simulink model "BATTERYLESS_SOLAR_INVERTER_DRIVE"  (R2021a)
settings: Solver=ode15s  StartTime=0.0  StopTime=inf  FixedStep=.00001  MaxStep=.00001  RelTol=1e-3  EnableMultiTasking=on
undefined symbols (not defined in the file): Capacitor, dEgdT, EgRef, gcbh, k1, Rsh_array5pc, Run, sps_rtmsupport, Start, Tref_K, VT_ref
libraries: fl_lib x7, spsCurrentMeasurementLib x6, nesl_utility x6, sh_lib x5, spsSeriesRLCBranchLib x5, spsIGBTDiodeLib x4, spsVoltageMeasurementLib x4, pid_lib x3, spsPVarrayModel x3, simulink x3, spsControlledCurrentSourceLib x2, spsRMSLib x2
(part 1 of 5)
settings Model: NumberOfSteps=100000000  Creator=Mahbubur Rahman  LastModifiedBy=This PC
settings SolverCC: AlgebraicLoopSolver=LineSearch
settings DataIOCC: LimitDataPoints=on  SaveFormat=Array  ReturnWorkspaceOutputs=off
settings OptimizationCC: LifeSpan=inf
settings DebuggingCC: SFUnexpectedBacktrackingDiag=warning  SFNoUnconditionalDefaultTransitionDiag=warning  SFExecutionAtInitializationDiag=none  SFMachineParentedDataDiag=warning  ArithmeticOperatorsInVariantConditions=warning
settings HardwareCC: ProdBitPerPointer=32  ProdBitPerSizeT=32  ProdBitPerPtrDiffT=32  ProdLargestAtomicFloat=None  ProdIntDivRoundTo=Undefined  ProdEndianess=Unspecified  ProdWordSize=32  ProdHWDeviceType=32-bit Generic
settings ModelReferenceCC: PropagateSignalLabelsOutOfModel=off
settings SFSimCC: SimUseLocalCustomCode=off  CustomCodeUndefinedFunction=UseInterfaceOnly
settings RTWCC: RTWUseLocalCustomCode=off
settings CodeAppCC: StateflowObjectComments=on
settings GRTTargetCC: TargetLangStandard=C89/C90 (ANSI)
settings ConfigComp: CovMetricSettings=dw  CovSaveCumulativeToWorkspaceVar=on  CovSaveSingleToWorkspaceVar=on  CovExternalEMLEnable=off
settings SimscapeCC: SimscapeNormalizeSystem=off

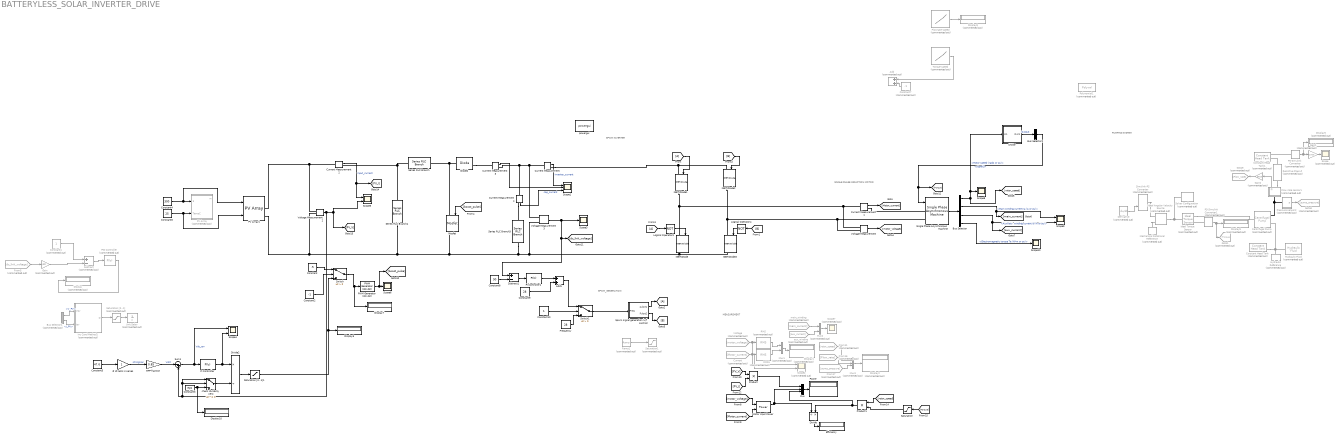
== system BATTERYLESS_SOLAR_INVERTER_DRIVE ==
  note: SPWM INVERTER
  note: PUMPING SYSTEM
  note: SINGLE PHASE INDUCTION MOTOR
  note: MEASUREMENT
  note: SPWM_GENERATION
  # of cells in series : Gain
  Add : Sum  Commented=on
  Add1 : Sum
  Bus Selector : BusSelector  OutputSignals="Mechanical.Rotor speed (rad/s or pu),Stator measurements.Main winding current Ia (A or pu),Stator measurements.Auxiliary  winding current Ib (A or pu),Mechanical.Electromagnetic torque Te (N*m or pu)"
  Bus Selector1 : BusSelector  Commented=on  OutputSignals=V_PV,I_PV
  Bus Selector2 : BusSelector  OutputSignals=signal3
  Centrifugal Pump : sh_lib/Pumps and Motors/Centrifugal Pump  Commented=on  mdl_type=1  c_1=326.8 Pa/(kg/m^3)  c_2=3.104e+4 Pa*s/kg  c_3=1.097e+7 Pa*s^2/(kg*m^3)  c_4=2.136e+5 Pa*s^2/(kg*m^3)  c_f=0.8  design_del=130 lpm  ref_velocity=1500 rpm  ref_density=1000 kg/m^3  leak_resistance=1e+8 Pa/(m^3/s)  T_const=0.1 N*m  trq_press_coeff=1e-6 N*m/Pa  pump_del_1D=[ 0 28 90 130 154 182 ] lpm  press_diff_1D=[ 2.6 2.4 2 1.6 1.2 0.8 ] bar  pump_del_power_1D=[ 0 20 40 60 80 100 120 140 160 ] lpm  power_1D=[ 220 280 310 360 390 420 480 500 550 ] W  pump_vel_2D=[ 3.2e+3 3.3e+3 3.4e+3 3.5e+3 ] rpm  pump_del_2D=[ 0 50 100 150 200 250 300 350 ] lpm  press_diff_2D=[ 8.300000000000001 8.800000000000001 9.300000000000001 9.9; 7.8 8.300000000000001 8.800000000000001 9.4; 7.2 7.6 8.199999999999999 8.699999999999999; 6.5 7 7.5 8; 5.6 6.1 6.6 7.1; 4.7 5.2 5.7 6.2; 3.4 4 4.4 4.9; 2.3 2.7 3.4 3.6 ] bar  pump_del_power_2D=[ 0 50 100 150 200 250 300 350 ] lpm  power_2D=[ 1.223e+3 1.341e+3 1.467e+3 1.6e+3; 1.414e+3 1.551e+3 1.696e+3 1.85e+3; 1.636e+3 1.794e+3 1.962e+3 2.14e+3; 1.941e+3 2.129e+3 2.326e+3 2.54e+3; 2.224e+3 2.439e+3 2.66e+3 2.91e+3; 2.453e+3 2.691e+3 2.947e+3 3.21e+3; 2.757e+3 3.024e+3 3.307e+3 3.608e+3; 2.945e+3 3.23e+3 3.533e+3 3.854e+3 ] W  omega_threshold=1e-9 rad/s  interp_method=2  extrap_method=1
      settings: SourceProductBaseCode=SH  InternalSimscapePortConfiguration="{\"Bottom\":[],\"Left\":[{\"id\":\"S\",\"label\":\"S\",\"type\":\"foundation.mechanical.rotational.rotational\"}],\"Right\":[{\"id\":\"P\",\"label\":\"P\",\"type\":\"foundation.hydraulic.hydraulic\"},{\"id\":\"T\",\"label\":\"T\",\"type\":\"foundation.hydraulic.hydraulic\"}],\"Top\":[]}"
  Chiller : Subsystem
  Constant : Constant  Value=.5
  Constant Head Tank : sh_lib/Low-Pressure Blocks/Constant Head Tank  Commented=on  press=0 Pa  fluid_level=1 m  pipe_diam=10 cm  loss_coeff=1.2  g=9.80665 m/s^2  volume_specify=on  volume_priority=High  volume=10000000 m^3  volume_nominal_specify=off  volume_nominal_unit=m^3  volume_nominal_value=1
      settings: SourceProductBaseCode=SH  InternalSimscapePortConfiguration="{\"Bottom\":[],\"Left\":[],\"Right\":[{\"id\":\"V\",\"label\":\"V\",\"type\":\"output\"},{\"id\":\"T\",\"label\":\"T\",\"type\":\"foundation.hydraulic.hydraulic\"}],\"Top\":[]}"
  Constant Head Tank1 : sh_lib/Low-Pressure Blocks/Constant Head Tank  Commented=on  press=0 Pa  fluid_level=0 m  pipe_diam=0.02 m  loss_coeff=1.2  g=9.80665 m/s^2  volume_specify=on  volume_priority=High  volume=0 m^3  volume_nominal_specify=off  volume_nominal_unit=m^3  volume_nominal_value=1
      settings: SourceProductBaseCode=SH  InternalSimscapePortConfiguration="{\"Bottom\":[],\"Left\":[],\"Right\":[{\"id\":\"V\",\"label\":\"V\",\"type\":\"output\"},{\"id\":\"T\",\"label\":\"T\",\"type\":\"foundation.hydraulic.hydraulic\"}],\"Top\":[]}"
  Constant1 : Constant  Commented=on
  Constant10 : Constant
  Constant2 : Constant  Value=-1
  Constant3 : Constant  Value=eps
  Constant4 : Constant  Value=300
  Constant5 : Constant  Value=47.6
  Constant6 : Constant  Value=25
  Constant7 : Constant  Commented=on  Value=.1
  Constant8 : Constant  Value=90
  Constant9 : Constant  Value=28
  Current : From  Commented=on  GotoTag=Motor_current
  Current Measurement{,1..4} (5 alike) : spsCurrentMeasurementLib/Current Measurement  PhasorSimulation=off  OutputType=Complex  PSBequivalent=0
  Derivative : Derivative  Commented=on
  Diode2 : spsDiodeLib/Diode  Ron=0.001  Lon=0  Vf=0.8  IC=0  UseSnubber=0  Rs=500  Cs=250e-9  Measurements=on
  Display{,1..2,6,8..9} (6 alike) : Display  Commented=on
  Display10 : Display
  Display5 : Display
  Display7 : Display
  Divide : Product  Inputs=/*
  Divide2 : Product  Inputs=*/
  "Efficiency " : Display
  Flow rate sensor1 : Subsystem  Commented=on
      mask Display:
      | plot([141.749396522682;150.34840079814;159.942662684676;170.439784195567;181.738672312351;193.730512565863;206.299816979056;219.32553627935;232.6822256693;246.241252928572;259.872037212541;273.443306617208;286.824362399395;299.886337677091;312.503438487969;324.554155254012;335.922432985171;346.498788952362;356.181367065997;364.876918805806;365.635077753444], [311.772266015396;301.195910048205;291.51333193457;282.817780194761;275.192997745505;268.712415409918;263.438444738539;259.421876951977;256.701393793698;255.303195003683;255.240746000613;256.514648202526;259.112633234831;263.009681081464;268.168261041319;274.538693169416;282.05962672193;290.658630997388;300.252892883924;310.750014394814;311.772273468441])
      | plot([141.699510299516;151.06208312931;161.43851880176;172.728886569004;184.8244540175;197.608734220609;210.958607571377;224.745507491653;238.836658598519;253.096355403808;267.387269232142;281.571770771148;295.513255516966;309.077459350303;322.133751573297;334.556392954544;346.225746666638;357.029430454211;366.863398936497;369.389910236765], [142.635753971168;153.439437758742;163.273406241027;172.042952925747;179.663622284404;186.062023105194;191.17653529049;194.957903292072;197.369710468977;198.388729799666;198.005147570929;196.222657889318;193.058427104875;188.542928489797;182.719648764172;175.644669295084;167.3861260024;158.023553172606;147.647117500155;144.622762828085])
      | plot([255.112000578148;241.220263814025;227.462288078042;213.97057019741;200.875042790642;188.30182294541;176.371997642044;165.200457619721;154.894790915842;145.554246734416;137.268779621969;130.118183156093;124.171321489666;119.485466151423;116.10574448982;114.064705072001;113.382004223305;114.064216726109;116.104772501074;119.484019880607;124.169414865158;130.115834539728;137.266011632208;145.551086028513;154.891267933124;165.196606288436;176.367855052617;188.297428993243;200.870439791896;213.965802481478;227.457401560637;241.21530555498;255.107018328207;268.99875509233;282.756730828313;296.248448708946;309.343976115713;321.917195960945;333.847021264311;345.018561286634;355.324227990513;364.66477217194;372.950239284386;380.100835750262;386.047697416689;390.733552754932;394.113274416535;396.154313834354;396.83701468305;396.154802180246;394.114246405281;390.734999025748;386.049604041197;380.103184366627;372.953007274147;364.667932877842;355.327750973232;345.022412617919;333.851163853738;321.921589913113;309.34857911446;296.253216424877;282.761617345719;269.003713351376;255.112000578149;255.112000578148;255.112000578148], [85.0365031729522;85.7187156757559;87.7592714507213;91.138518830254;95.823913814805;101.770333489375;108.920510581855;117.20558497816;126.54576688277;136.851105238083;148.022354002264;159.951927942889;172.524938741542;185.620301431125;199.111900510283;212.869804504627;226.761517277854;240.653254041976;254.41122977796;267.902947658592;280.99847506536;293.571694910592;305.501520213958;316.673060236281;326.97872694016;336.319271121586;344.604738234033;351.755334699909;357.702196366336;362.388051704579;365.767773366182;367.808812784001;368.491513632697;367.809301129893;365.768745354927;362.389497975395;357.704102990844;351.757683316273;344.607506223793;336.322431827489;326.982249922878;316.676911567566;305.505662803384;293.576088862759;281.003078064106;267.907715374523;254.416116295365;240.658212301022;226.766499527795;212.874762763672;199.116787027689;185.625069147057;172.529541740289;159.956321895057;148.026496591691;136.854956569369;126.54928986549;117.208745684063;108.923278571616;101.77268210574;95.8258204393135;91.1399651010703;87.7602434394666;85.7192040216476;85.0365031729522;85.0365031729522;85.0365031729522])
      | plot([113.382004201412;56.6910021007061], [226.764008402824;226.764008402824])
      | plot([396.837014704943;453.528016805649;450.693466700613], [226.764008402824;226.764008402824;226.764008402824])
      | plot([510.219018906355;0;0;510.219018906355;510.219018906355], [510.219018906355;510.219018906355;0;0;510.219018906355])
      | ;color('red');
      | port_label('LConn', 1,'A')
      | port_label('RConn', 1,'B')
  Flowrate-speed : Lookup_n-D  Commented=on  NumberOfTableDimensions=1  BreakpointsForDimension1=[0,0.755267129742124,3.94138541604345,4.4414537006491,7.53165396046033,8.07857474382879,11.1492675042464,11.7097698895216,14.7704457545395,15.3535511531923,18.3855000155405,19.023728886058,21.9935096148579,22.730877418348,25.6001483967937,26.4827517809723,29.2158883182174,30.283293810304,32.8535466181619,34.1309377359887,36.5253360532606,38.0175805064918,40.2403035353047,41.9296372251585,44.0030919829905,45.8517320387111,47.8142383144331,49.7719032061007,51.6711955449403,53.6857443686728,55.5689445180788,57.5970867055065,59.5000308517515,61.5149482189319,63.4551949595903,65.4488392003123,67.4256256724198,69.4050214570267,71.4059609943714,73.3849875878053,75.3957115737105,77.3860986863011,79.3978365933288,81.4038216961908,83.4156531732883,85.434477767689,87.4503871026008,89.4768321784884,91.5007566875217,93.5315546937149,95.5585766457447,96.3816078917583,97.1583244877688,97.5553159469706,98.5109556896585,98.942464160912,99.7574872364738,100.421283742859,101.07463594914,101.853778607577,102.481394416513,103.244540211763,103.936132120085,104.652018040325,105.393813499244,106.098856898837,106.848483926202,107.575303616505,108.316989524379,109.066251289772,109.809284913161,110.568387478049,111.323498843144,112.086670722946,112.854874120687,113.624667016258,114.40227865717,115.182041566037,115.967331307467,116.757422142148,117.551245116694,118.350605567398,119.153989085531,119.962222924494,120.775257982183,121.592720182895,122.415140879025,123.242160081895,124.073946581288,124.910563281961,125.751889693993,126.598080049304,127.449074625766,128.304901941835,129.165610952387,130.031176064865,130.90164360049,131.777020135967,132.657315099945,133.542556003384,134.432747653115,135.327908481052,136.228053440758,137.133192405713,138.043341260578,138.958510842986,139.87871256473,140.803958431303,141.734257902805,142.669621071515,143.610056994698,144.555573622054,145.50617867552,146.461878717645,147.422679531354,148.38858614358,149.359602511583,150.335731721296,151.316975860531,152.30333593763,153.294811920063,154.291402633151,155.293105725223,156.299917638184,157.311833536082,158.328847265387,159.350951303764,160.378136699555,161.410393021146,162.447708298236,163.490068961237,164.537459782067,165.589863810492,166.647262309323,167.709634688423,168.776958435952,169.849206150296,170.923006726351,171.99390815586,173.062561647706,174.129436376986,175.194952410275,176.259419194953,177.323066108992,178.386056645792,179.448487812122,180.510448409105,181.572036759616,182.633352690859,183.694493078604,184.755547514223,185.816595543058,186.877705530537,187.93893392239,189.000325086927,190.061911650665,191.123715182272,192.185758808865,193.248076932833,194.310686031143,195.373582867113,196.436747999436,197.500148410283,198.563739469472,199.627466414353,200.6912655164,201.755065006481,202.818785812219,203.882342160934,204.945642078165,206.008587802641,207.071076137412,208.132998750829,209.19424243718,210.254689345506,211.31421718332,212.372699400335,213.430005356484,214.486000477789,215.540546402947,216.59350112303,217.644719116346,218.694051480172,219.741346060803,220.786448265843,221.829205247654,222.869465287781,223.907074945561,224.941879059511,225.973720793947,227.002441697075,228.027881769757,229.049879541202,230.06827215286,231.08289545147,232.093584090637,233.100171640738,234.102490707285,235.100373057609,236.093649755654,237.082151304686,238.065707797705,239.044149075298,240.017304890621,240.985005081183,241.947079747063,242.903359435172,243.853675329111,244.797859444178,245.735744827019,246.6671657594,247.591957965548,248.50995882248,249.421007572714,250.32494553873,251.221616338524,252.110866101598,252.99254368468,253.86650088649,254.732592660822,255.590677327237,256.440616778643,257.28227668503,258.115526692641,258.940240617881,259.756296635252,260.563577458626,261.36197051521,262.15136811153,262.931667590861,263.702771481481,264.464587635229,265.217029355844,265.960015516618,266.693470666946,267.417325127393,268.131515072948 ...(+2740 chars)]  Table=[-2.49551596944865e-05,-2.49549147032931e-05,-2.49484380819495e-05,-2.49466297780723e-05,-2.49306026044872e-05,-2.49269113638027e-05,-2.49013121298883e-05,-2.48957594374241e-05,-2.48605733783786e-05,-2.48529407394126e-05,-2.480845080358e-05,-2.47980468706096e-05,-2.47449474830391e-05,-2.47305343651049e-05,-2.46699144918519e-05,-2.46497599560278e-05,-2.45829899241857e-05,-2.45550454605781e-05,-2.4483588126165e-05,-2.44457860626406e-05,-2.43709488524717e-05,-2.4321576461125e-05,-2.42442283291449e-05,-2.41822885846768e-05,-2.41025904730598e-05,-2.40280252732902e-05,-2.3945261125573e-05,-2.38589273594273e-05,-2.37715467273756e-05,-2.36749127185171e-05,-2.35808557660346e-05,-2.34754954913822e-05,-2.33727420647344e-05,-2.32597916187635e-05,-2.31469168499245e-05,-2.30266881082214e-05,-2.29031464467343e-05,-2.27750597666361e-05,-2.2641042316839e-05,-2.25039266552064e-05,-2.23598806835534e-05,-2.22124971407542e-05,-2.20585923775605e-05,-2.19000743546397e-05,-2.17359181246507e-05,-2.1565859764012e-05,-2.13905911859891e-05,-2.12087761130309e-05,-2.10214053780375e-05,-2.08274350068393e-05,-2.06276763071934e-05,-2.0544708332486e-05,-2.04655251262348e-05,-2.04246356753725e-05,-2.03253729585894e-05,-2.02799850665838e-05,-2.01935869076218e-05,-2.01223720606876e-05,-2.0051575766443e-05,-1.99662400392406e-05,-1.98967224332311e-05,-1.98113241626112e-05,-1.97330411005835e-05,-1.96511354611788e-05,-1.95653090927907e-05,-1.94828100497838e-05,-1.93941129044323e-05,-1.930711683095e-05,-1.92173274242324e-05,-1.91255616966952e-05,-1.90334902991678e-05,-1.89383183557908e-05,-1.88425118100022e-05,-1.87445187791029e-05,-1.86446778313321e-05,-1.85434008084471e-05,-1.84398264912865e-05,-1.83346618978678e-05,-1.82274108267435e-05,-1.81181212626141e-05,-1.80068930196575e-05,-1.78934217523123e-05,-1.77778671345495e-05,-1.76600553422711e-05,-1.75399336130264e-05,-1.74174959571178e-05,-1.72925985157255e-05,-1.71652278871072e-05,-1.70352876409391e-05,-1.69026932578763e-05,-1.67673856293163e-05,-1.66292577592988e-05,-1.64882325221105e-05,-1.63442138742351e-05,-1.61970969820236e-05,-1.60467841169421e-05,-1.58931592194649e-05,-1.57361065042925e-05,-1.55755026505602e-05,-1.54112132679794e-05,-1.52430996363834e-05,-1.50710112360041e-05,-1.48947879668254e-05,-1.47142594923345e-05,-1.45292418833336e-05,-1.43395384646981e-05,-1.41449371791413e-05,-1.39452088002874e-05,-1.37401055714289e-05,-1.3529358168955e-05,-1.33126733045148e-05,-1.30897305185023e-05,-1.28601781590027e-05,-1.26236290618357e-05,-1.2379655032421e-05,-1.21277802855679e-05,-1.18674735560113e-05,-1.15981382649136e-05,-1.13191004222428e-05,-1.10295934435953e-05,-1.07287388420761e-05,-1.04155214338913e-05,-1.00887569265338e-05,-9.74704884365562e-06,-9.38873016383182e-06,-9.01178241294498e-06,-8.61372054797799e-06,-8.19142403767303e-06,-7.74087967555675e-06,-7.25677202315763e-06,-6.73179360231919e-06,-6.15539614279133e-06,-5.51130007439783e-06,-4.7717907156445e-06,-3.88146314991264e-06,-2.68623152633747e-06,1.25160354243976,63.3665222781476,119.652343191978,171.805480489557,220.121632951326,265.161240746742,307.558847273221,347.779385477827,386.506555351731,424.189316880001,460.699631721232,495.965114144391,529.961450844176,562.700870365115,594.221157898742,624.576449882164,653.830146784885,682.049771150408,709.303441601163,735.657585852094,761.16848729897,785.802243671772,809.653445329318,832.838381314817,855.448629118332,877.557723581626,899.225678657012,920.502149201249,941.428700665877,962.040476456674,982.367447082747,1002.43536223163,1022.26648778397,1041.88018419473,1061.2933659522,1080.52087066198,1099.57575853552,1118.46955763738,1137.21246641651,1155.81352226635,1174.28074282024,1192.62124518544,1210.84134719072,1228.94665386502,1246.94213171072,1264.83217282952,1282.62065056483,1300.31096801495,1317.90063638302,1335.37823672611,1352.74020310878,1369.98343411612,1387.10503185905,1404.1022908572,1420.97268689659,1437.7138659716,1454.32363335805,1470.79994293292,1487.14088683621,1503.3446855316 ...(+3432 chars)]  InternalRulePriority=Speed  RndMeth=Simplest  InputSameDT=on
  "Frequency " : Constant  Value=28
  From11 : From  Commented=on  GotoTag=rotor_speed
  From16 : From  Commented=on  GotoTag=Flow_rate
  From17 : From  Commented=on  GotoTag=pump_pressure
  From5 : From  Commented=on  GotoTag=dc_link_voltage
  Gain : Gain  Commented=on  Gain=1/80
  Gain1 : Gain  Commented=on  Gain=1000
  Gain2 : Gain  Commented=on  Gain=36e5
  Goto1 : Goto  Commented=on  GotoTag=Torque
  Goto8 : Goto  Commented=on  GotoTag=pump_pressure
  Goto9 : Goto  Commented=on  GotoTag=Flow_rate
  Hydraulic Fluid : sh_lib/Hydraulic Utilities/Hydraulic Fluid  Commented=on  DataSource=1  SelFluid=24  SysTemp=60  TrapAir=0.005  ViscDerFactor=1  range_error=2
  Hydraulic Reference : fl_lib/Hydraulic/Hydraulic Elements/Hydraulic Reference  Commented=on
  IGBT/Diode{,1..3} (4 alike) : spsIGBTDiodeLib/IGBT//Diode  Ron=1e-3  Rs=1e5  Cs=inf  Measurements=on
  Ideal Angular Velocity Source : fl_lib/Mechanical/Mechanical Sources/Ideal Angular Velocity Source  Commented=on
  Ideal Torque Sensor : fl_lib/Mechanical/Mechanical Sensors/Ideal Torque Sensor  Commented=on
  Inc Cond Method1 : Stateflow chart  Commented=on  TreatAsAtomicUnit=on
  Logical Operator3 : Logic  Operator=NOT  AllPortsSameDT=off  OutDataTypeStr=boolean
  Logical Operator4 : Logic  Operator=NOT  AllPortsSameDT=off  OutDataTypeStr=boolean
  MPP fraction : Gain  Gain=0.85
  Mechanical Rotational Reference : fl_lib/Mechanical/Rotational Elements/Mechanical Rotational Reference  Commented=on
  Mosfet : spsMosfetLib/Mosfet  Ron=1e-3  Lon=0  Rd=1e-3  Vfd=0  IC=0  Rs=1e5  Cs=inf  Measurements=on
  Motor Input Power : spsPowerLib/Power  Freq=19  Vinit=[1, 0]  Iinit=[1, 0]  Ts=0
      settings: SourceProductBaseCode=PS
  Mux : Mux  Inputs=3
  Mux1 : Mux  Commented=on  Inputs=2
  Mux2 : Mux  Commented=on  Inputs=2
  Mux3 : Mux  Commented=on  Inputs=3
  PI Controller : pid_lib/PID Controller  Controller=PI  Form=Parallel  TimeDomain=Discrete-time  UseExternalTs=off  SampleTime=1e-4  IntegratorMethod=Forward Euler  FilterMethod=Forward Euler  ControllerParametersSource=internal  P=1  I=50  D=0  UseFilter=on  N=100  TunerSelectOption=Transfer Function Based (PID Tuner App)  ZeroCross=off  InitialConditionSource=internal  InitialConditionForIntegrator=0  InitialConditionForFilter=0  DifferentiatorICPrevScaledInput=0  ExternalReset=none  TrackingMode=off  Kt=1  LimitOutput=on  SatLimitsSource=internal  UpperSaturationLimit=36  LowerSaturationLimit=-4  LinearizeAsGain=off  AntiWindupMode=clamping  Kb=20  POutMin=[]  POutMax=[]  IOutMin=[]  IOutMax=[]  DOutMin=[]  DOutMax=[]  NOutMin=[]  NOutMax=[]  SumOutMin=[]  SumOutMax=[]  SaturationOutMin=[]  SaturationOutMax=[]  PParamMin=[]  PParamMax=[]  IParamMin=[]  IParamMax=[]  DParamMin=[]  DParamMax=[]  NParamMin=[]  NParamMax=[]  KbParamMin=[]  KbParamMax=[]  KtParamMin=[]  KtParamMax=[]  KbOutMin=[]  KbOutMax=[]  KtOutMin=[]  KtOutMax=[]  IntegratorOutMin=[]  IntegratorOutMax=[]  FilterOutMin=[]  FilterOutMax=[]  SumI1OutMin=[]  SumI1OutMax=[]  SumI2OutMin=[]  SumI2OutMax=[]  SumI3OutMin=[]  SumI3OutMax=[]  SumI4OutMin=[]  SumI4OutMax=[]  SumDOutMin=[]  SumDOutMax=[]  DifferentiatorOutMin=[]  DifferentiatorOutMax=[]  FilterDiffOutCoefMin=[]  FilterDiffOutCoefMax=[]  ReciprocalOutMin=[]  ReciprocalOutMax=[]  SumDenOutMin=[]  SumDenOutMax=[]  SumNumOutMin=[]  SumNumOutMax=[]  DivideOutMin=[]  DivideOutMax=[]  UdiffTsProdOutMin=[]  UdiffTsProdOutMax=[]  NTsProdOutMin=[]  NTsProdOutMax=[]  UintegralTsProdOutMin=[]  UintegralTsProdOutMax=[]  UngainTsProdOutMin=[]  UngainTsProdOutMax=[]  IntegratorContinuousStateAttributes=''  IntegratorStateMustResolveToSignalObject=off  IntegratorRTWStateStorageClass=Auto  FilterContinuousStateAttributes=''  FilterStateMustResolveToSignalObject=off  FilterRTWStateStorageClass=Auto  ParallelPVariant=InternalParameters  IdealPVariant=Disabled  IVariant=InternalParameters  DVariant=Disabled  IntegratorVariant=Discrete  SatVariant=Enabled  AWVariant=DiscClampingParallel  PCopyVariant=Disabled  TRVariant=Disabled  FdbkBlocksVariant=Forward  IdealPFdbkVariant=Disabled  SatFdbkVariant=Disabled  DerivativeFilterVariant=Disabled  NVariant=Disabled  NCopyVariant=Disabled_SignalSpec  FilterICVariant=Disabled  IntegratorICVariant=InternalICs  ExternalResetVariant=Disabled  TRSumVariant=Passthrough  SumFdbkVariant=Disabled  SumVariant=Sum_PI  TsampFilterVariant=InternalTs  TsampNgainVariant=Passthrough  TsampIntegralVariant=Passthrough  ExternalSaturationOutDataTypeStr=Inherit: Same as second input
  PI Controller1 : pid_lib/PID Controller  Controller=PI  Form=Parallel  TimeDomain=Discrete-time  UseExternalTs=off  SampleTime=1e-4  IntegratorMethod=Forward Euler  FilterMethod=Forward Euler  ControllerParametersSource=internal  P=.1  I=20  D=0  UseFilter=on  N=100  TunerSelectOption=Transfer Function Based (PID Tuner App)  ZeroCross=off  InitialConditionSource=internal  InitialConditionForIntegrator=0  InitialConditionForFilter=0  DifferentiatorICPrevScaledInput=0  ExternalReset=none  TrackingMode=off  Kt=1  LimitOutput=on  SatLimitsSource=internal  UpperSaturationLimit=36  LowerSaturationLimit=-10  LinearizeAsGain=off  AntiWindupMode=clamping  Kb=20  POutMin=[]  POutMax=[]  IOutMin=[]  IOutMax=[]  DOutMin=[]  DOutMax=[]  NOutMin=[]  NOutMax=[]  SumOutMin=[]  SumOutMax=[]  SaturationOutMin=[]  SaturationOutMax=[]  PParamMin=[]  PParamMax=[]  IParamMin=[]  IParamMax=[]  DParamMin=[]  DParamMax=[]  NParamMin=[]  NParamMax=[]  KbParamMin=[]  KbParamMax=[]  KtParamMin=[]  KtParamMax=[]  KbOutMin=[]  KbOutMax=[]  KtOutMin=[]  KtOutMax=[]  IntegratorOutMin=[]  IntegratorOutMax=[]  FilterOutMin=[]  FilterOutMax=[]  SumI1OutMin=[]  SumI1OutMax=[]  SumI2OutMin=[]  SumI2OutMax=[]  SumI3OutMin=[]  SumI3OutMax=[]  SumI4OutMin=[]  SumI4OutMax=[]  SumDOutMin=[]  SumDOutMax=[]  DifferentiatorOutMin=[]  DifferentiatorOutMax=[]  FilterDiffOutCoefMin=[]  FilterDiffOutCoefMax=[]  ReciprocalOutMin=[]  ReciprocalOutMax=[]  SumDenOutMin=[]  SumDenOutMax=[]  SumNumOutMin=[]  SumNumOutMax=[]  DivideOutMin=[]  DivideOutMax=[]  UdiffTsProdOutMin=[]  UdiffTsProdOutMax=[]  NTsProdOutMin=[]  NTsProdOutMax=[]  UintegralTsProdOutMin=[]  UintegralTsProdOutMax=[]  UngainTsProdOutMin=[]  UngainTsProdOutMax=[]  IntegratorContinuousStateAttributes=''  IntegratorStateMustResolveToSignalObject=off  IntegratorRTWStateStorageClass=Auto  FilterContinuousStateAttributes=''  FilterStateMustResolveToSignalObject=off  FilterRTWStateStorageClass=Auto  ParallelPVariant=InternalParameters  IdealPVariant=Disabled  IVariant=InternalParameters  DVariant=Disabled  IntegratorVariant=Discrete  SatVariant=Enabled  AWVariant=DiscClampingParallel  PCopyVariant=Disabled  TRVariant=Disabled  FdbkBlocksVariant=Forward  IdealPFdbkVariant=Disabled  SatFdbkVariant=Disabled  DerivativeFilterVariant=Disabled  NVariant=Disabled  NCopyVariant=Disabled_SignalSpec  FilterICVariant=Disabled  IntegratorICVariant=InternalICs  ExternalResetVariant=Disabled  TRSumVariant=Passthrough  SumFdbkVariant=Disabled  SumVariant=Sum_PI  TsampFilterVariant=InternalTs  TsampNgainVariant=Passthrough  TsampIntegralVariant=Passthrough  ExternalSaturationOutDataTypeStr=Inherit: Same as second input
  PID Controller : pid_lib/PID Controller  Commented=on  Controller=PI  Form=Parallel  TimeDomain=Continuous-time  UseExternalTs=off  SampleTime=-1  IntegratorMethod=Forward Euler  FilterMethod=Forward Euler  ControllerParametersSource=internal  P=.7  I=30  D=0  UseFilter=on  N=100  TunerSelectOption=Transfer Function Based (PID Tuner App)  InitialConditionSource=internal  InitialConditionForIntegrator=0  InitialConditionForFilter=0  DifferentiatorICPrevScaledInput=0  ExternalReset=none  TrackingMode=off  Kt=1  LimitOutput=on  SatLimitsSource=internal  UpperSaturationLimit=.9  LowerSaturationLimit=.1  LinearizeAsGain=on  AntiWindupMode=none  Kb=1  POutMin=[]  POutMax=[]  IOutMin=[]  IOutMax=[]  DOutMin=[]  DOutMax=[]  NOutMin=[]  NOutMax=[]  SumOutMin=[]  SumOutMax=[]  SaturationOutMin=[]  SaturationOutMax=[]  PParamMin=[]  PParamMax=[]  IParamMin=[]  IParamMax=[]  DParamMin=[]  DParamMax=[]  NParamMin=[]  NParamMax=[]  KbParamMin=[]  KbParamMax=[]  KtParamMin=[]  KtParamMax=[]  KbOutMin=[]  KbOutMax=[]  KtOutMin=[]  KtOutMax=[]  IntegratorOutMin=[]  IntegratorOutMax=[]  FilterOutMin=[]  FilterOutMax=[]  SumI1OutMin=[]  SumI1OutMax=[]  SumI2OutMin=[]  SumI2OutMax=[]  SumI3OutMin=[]  SumI3OutMax=[]  SumI4OutMin=[]  SumI4OutMax=[]  SumDOutMin=[]  SumDOutMax=[]  DifferentiatorOutMin=[]  DifferentiatorOutMax=[]  FilterDiffOutCoefMin=[]  FilterDiffOutCoefMax=[]  ReciprocalOutMin=[]  ReciprocalOutMax=[]  SumDenOutMin=[]  SumDenOutMax=[]  SumNumOutMin=[]  SumNumOutMax=[]  DivideOutMin=[]  DivideOutMax=[]  UdiffTsProdOutMin=[]  UdiffTsProdOutMax=[]  NTsProdOutMin=[]  NTsProdOutMax=[]  UintegralTsProdOutMin=[]  UintegralTsProdOutMax=[]  UngainTsProdOutMin=[]  UngainTsProdOutMax=[]  IntegratorContinuousStateAttributes=''  IntegratorStateMustResolveToSignalObject=off  IntegratorRTWStateStorageClass=Auto  FilterContinuousStateAttributes=''  FilterStateMustResolveToSignalObject=off  FilterRTWStateStorageClass=Auto  ParallelPVariant=InternalParameters  IdealPVariant=Disabled  IVariant=InternalParameters  DVariant=Disabled  IntegratorVariant=Continuous  SatVariant=Enabled  AWVariant=Passthrough  PCopyVariant=Disabled  TRVariant=Disabled  FdbkBlocksVariant=Forward  IdealPFdbkVariant=Disabled  SatFdbkVariant=Disabled  DerivativeFilterVariant=Disabled  NVariant=Disabled  NCopyVariant=Disabled_SignalSpec  FilterICVariant=Disabled  IntegratorICVariant=InternalICs  ExternalResetVariant=Disabled  TRSumVariant=Passthrough  SumFdbkVariant=Disabled  SumVariant=Sum_PI  TsampFilterVariant=InternalTs  TsampNgainVariant=Passthrough  TsampIntegralVariant=Passthrough  ExternalSaturationOutDataTypeStr=Inherit: Same as second input
  PS-Simulink Converter : nesl_utility/PS-Simulink Converter  Commented=on  PhysicalDomain=network_engine_domain  SubClassName=ps_output  LeftPortType=input  RightPortType=output  PseudoPeriodic=off  Frequencies=[]  Unit=1  AffineConversion=off
      settings: SourceProductBaseCode=PW,SS
  PS-Simulink Converter1 : nesl_utility/PS-Simulink Converter  Commented=on  PhysicalDomain=network_engine_domain  SubClassName=ps_output  LeftPortType=input  RightPortType=output  PseudoPeriodic=off  Frequencies=[]  Unit=N*m  AffineConversion=off
      settings: SourceProductBaseCode=PW,SS
  PV Array : Subsystem  Commented=on  AncestorBlock=re_lib/Solar/PV Array  DialogController=POWERSYS.PowerSysDialog  LoadFcn=sps_rtmsupport('LoadFcn',gcbh);  StartFcn=sps_rtmsupport('StartFcn',gcbh);  StopFcn=sps_rtmsupport('StopFcn',gcbh);  mask(PV array){Npar=1, Nser=2, PlotType=array @ 25 deg.C & specified irradiances, S_vec=[350 500 800], Temp_C_vec=[ 45 25  ], ModuleName=User-defined, PlotWhenSelected=off, Pm=61.425, Ncell=60, Voc=21.5, Isc=3.95, Vm=17.5, Im=3.51, beta_Voc_pc=-0.36099, alpha_Isc_pc=0.102, beta_Voc=-0.077613, alpha_Isc=0.004029, IL=3.9807, I0=1.4561e-10, nI=0.5825, Rsh=64.1721, Rs=0.37085, BAL=off, Tc=1e-6, Tfilter=5e-5}
      mask prompts: Npar "Parallel strings"; Nser "Series-connected modules per string"; S_vec "Irradiances (W/m2)"; Temp_C_vec "T_cell (deg. C)"; ModuleName "Module:"; PlotWhenSelected "Plot I-V and P-V characteristics when a module is selected"; Pm "Maximum Power (W)"; Ncell "Cells per module (Ncell)"; Voc "Open circuit voltage  Voc (V)"; Isc "Short-circuit current Isc (A)"; Vm "Voltage at maximum power point Vmp (V)"; Im "Current at maximum power point Imp (A)"; beta_Voc_pc "Temperature coefficient of Voc (%/deg.C)"; alpha_Isc_pc "Temperature coefficient of Isc (%/deg.C)"; beta_Voc "Temperature coefficient of Voc (V/deg.C)"; alpha_Isc "Temperature coefficient of Isc (A/deg.C)"; IL "Light-generated current IL (A)"; I0 "Diode saturation current I0 (A)"; nI "Diode ideality factor"; Rsh "Shunt resistance Rsh (ohms)"; Rs "Series resistance Rs (ohms)"; BAL "Break algebaic loop in internal model"; Tc "Time constant (s)"; Tfilter "Time constant (s)"
      mask help:
      | Implements a PV array built of strings of PV modules connected in parallel. Each string consists of modules connected in series.
      | Allows modeling of a variety of preset PV modules available from NREL System Advisor Model (Jan. 2014) as well as user-defined PV module.
      |
      | Input 1 = Sun irradiance, in W/m2, and input 2 = Cell temperature, in deg.C.
      mask init:
      | Block = gcb;
      | [k,k1,q,Tref_C,Tref_K,EgRef,dEgdT,Rsh_array5pc,VT_ref,Tsf,Tf,WantBlockChoice] = PVArrayInit(Block, ModuleName, Nser, Npar, Ncell, Rsh, nI, Tfilter);
      | powericon('SetInternalModels','set',Block,WantBlockChoice);
      | sps_rtmsupport('parametereditingmodes',Block, [3 6 7 23]);
      settings: CopyFcn=sps_rtmsupport('CopyFcn',gcbh);  DeleteFcn=sps_rtmsupport('DeleteFcn',gcbh);  UndoDeleteFcn=sps_rtmsupport('UndoDeleteFcn',gcbh);  ModelCloseFcn=sps_rtmsupport('ModelCloseFcn',gcbh);  PreSaveFcn=sps_rtmsupport('PreSaveFcn',gcbh);  PostSaveFcn=sps_rtmsupport('PostSaveFcn',gcbh);  NameChangeFcn=sps_rtmsupport('NameChangeFcn',gcbh);  PreCopyFcn=sps_rtmsupport('PreCopyFcn',gcbh);  CloseFcn=sps_rtmsupport('CloseFcn',gcbh);  PreDeleteFcn=sps_rtmsupport('PreDeleteFcn',gcbh);
      settings: OpenFcn=|
      | %assignin('base','PVMaskOpening',1);
      | %open_system(gcb,'mask')
      | %assignin('base','PVMaskOpening',0);
      | sps_rtmsupport('OpenFcn',gcbh, [3 6 7 23]);
      mask Help: helpview(psbhelp);
      mask TypeOptions PlotType: one module @ 25 deg.C & specified irradiances | array @ 25 deg.C & specified irradiances | array @ 1000 W/m2 & specified temperatures
      mask Callback PlotType: PVArrayCback(gcb)
